simulink library "GTM_aerolib"  (Simulink 7.2)
settings: Solver=ode45  SolverMode=SingleTasking  StartTime=0.0  StopTime=10.0  RelTol=1e-3
undefined symbols (not defined in the file or in its folder): Aero, DamageModels
libraries: simulink_need_slupdate x58, GTM_aerolib x8, simulink x3
(part 3 of 3)

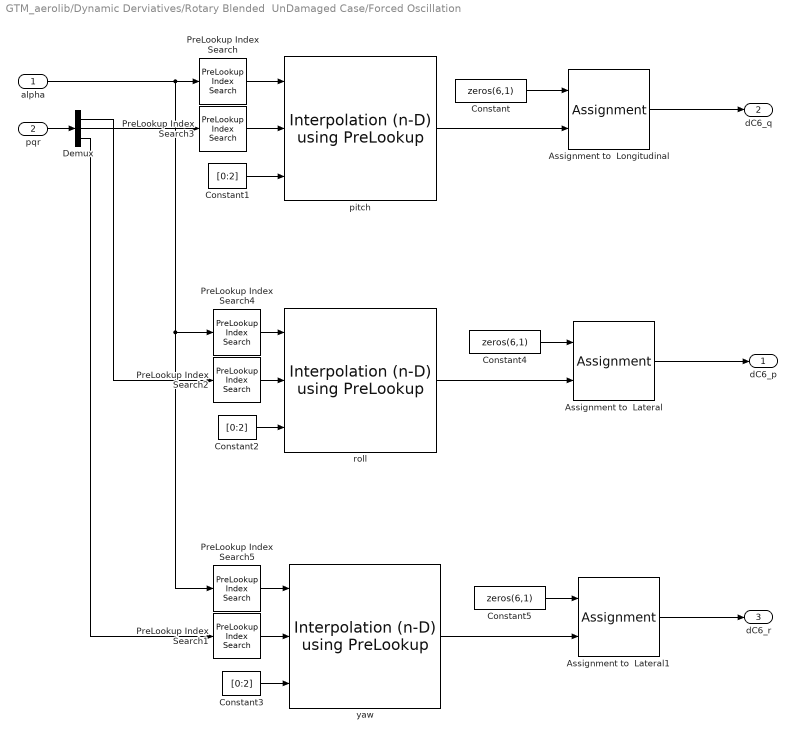
== system GTM_aerolib/Dynamic Derviatives/Rotary Blended  UnDamaged Case/Forced Oscillation ==
  alpha : Inport  OutDataType=sfix(16)  OutScaling=2^0
  pqr : Inport  Port=2  OutDataType=sfix(16)  OutScaling=2^0
  Assignment to  Lateral : Assignment  IndexMode=Zero-based  IndexOptions=Index vector (dialog)  Indices=[1 3 5]  OutputSizes=[1 1]
  Assignment to  Lateral1 : Assignment  IndexMode=Zero-based  IndexOptions=Index vector (dialog)  Indices=[1 3 5]  OutputSizes=[1 1]
  Assignment to  Longitudinal : Assignment  IndexMode=Zero-based  IndexOptions=Index vector (dialog)  Indices=[0 2 4]  OutputSizes=[1 1]
  Constant : Constant  Value=zeros(6,1)  OutDataType=sfix(16)  OutScaling=2^0
  Constant1 : Constant  Value=[0:2]  OutDataTypeMode=uint32  OutDataType=sfix(16)  OutScaling=2^0  OutDataTypeStr=uint32
  Constant2 : Constant  Value=[0:2]  OutDataTypeMode=uint32  OutDataType=sfix(16)  OutScaling=2^0  OutDataTypeStr=uint32
  Constant3 : Constant  Value=[0:2]  OutDataTypeMode=uint32  OutDataType=sfix(16)  OutScaling=2^0  OutDataTypeStr=uint32
  Constant4 : Constant  Value=zeros(6,1)  OutDataType=sfix(16)  OutScaling=2^0
  Constant5 : Constant  Value=zeros(6,1)  OutDataType=sfix(16)  OutScaling=2^0
  Demux : Demux  Outputs=3
  PreLookup Index Search : simulink_need_slupdate/PreLookup Index Search  bpData=Aero.dC3_q.alpha  searchMode=Binary Search  cacheBpFlag=on  outputFlag=off  IndexDataType=uint32  extrapMode=Linear Extrapolation  rangeErrorMode=None
  PreLookup Index Search1 : simulink_need_slupdate/PreLookup Index Search  bpData=Aero.dC3_r.rhat  searchMode=Binary Search  cacheBpFlag=on  outputFlag=off  IndexDataType=uint32  extrapMode=Linear Extrapolation  rangeErrorMode=None
  PreLookup Index Search2 : simulink_need_slupdate/PreLookup Index Search  bpData=Aero.dC3_p.phat  searchMode=Binary Search  cacheBpFlag=on  outputFlag=off  IndexDataType=uint32  extrapMode=Linear Extrapolation  rangeErrorMode=None
  PreLookup Index Search3 : simulink_need_slupdate/PreLookup Index Search  bpData=Aero.dC3_q.qhat  searchMode=Binary Search  cacheBpFlag=on  outputFlag=off  IndexDataType=uint32  extrapMode=Linear Extrapolation  rangeErrorMode=None
  PreLookup Index Search4 : simulink_need_slupdate/PreLookup Index Search  bpData=Aero.dC3_p.alpha  searchMode=Binary Search  cacheBpFlag=on  outputFlag=off  IndexDataType=uint32  extrapMode=Linear Extrapolation  rangeErrorMode=None
  PreLookup Index Search5 : simulink_need_slupdate/PreLookup Index Search  bpData=Aero.dC3_r.alpha  searchMode=Binary Search  cacheBpFlag=on  outputFlag=off  IndexDataType=uint32  extrapMode=Linear Extrapolation  rangeErrorMode=None
  pitch : simulink_need_slupdate/Interpolation (n-D) using PreLookup  numDimsPopupSelect=3  explicitNumDims=2  table=Aero.dC3_q.data  interpMethod=Linear  extrapMethod=Linear  rangeErrorMode=None  NumSelectionDims=1
  roll : simulink_need_slupdate/Interpolation (n-D) using PreLookup  numDimsPopupSelect=3  explicitNumDims=2  table=Aero.dC3_p.data  interpMethod=Linear  extrapMethod=Linear  rangeErrorMode=None  NumSelectionDims=1
  yaw : simulink_need_slupdate/Interpolation (n-D) using PreLookup  numDimsPopupSelect=3  explicitNumDims=2  table=Aero.dC3_r.data  interpMethod=Linear  extrapMethod=Linear  rangeErrorMode=None  NumSelectionDims=1
  dC6_p : Outport  OutDataType=sfix(16)  OutScaling=2^0
  dC6_q : Outport  Port=2  OutDataType=sfix(16)  OutScaling=2^0
  dC6_r : Outport  Port=3  OutDataType=sfix(16)  OutScaling=2^0
  wires:
  PreLookup Index Search5/1 -> yaw/1
  PreLookup Index Search4/1 -> roll/1
  PreLookup Index Search/1 -> pitch/1
  Assignment to  Longitudinal/1 -> dC6_q/1
  Assignment to  Lateral1/1 -> dC6_r/1
  Assignment to  Lateral/1 -> dC6_p/1
  PreLookup Index Search3/1 -> pitch/2
  PreLookup Index Search2/1 -> roll/2
  PreLookup Index Search1/1 -> yaw/2
  yaw/1 -> Assignment to  Lateral1/2
  Constant5/1 -> Assignment to  Lateral1/1
  Constant4/1 -> Assignment to  Lateral/1
  roll/1 -> Assignment to  Lateral/2
  pitch/1 -> Assignment to  Longitudinal/2
  Constant/1 -> Assignment to  Longitudinal/1
  Constant3/1 -> yaw/3
  Constant2/1 -> roll/3
  Demux/3 -> PreLookup Index Search1/1
  Demux/1 -> PreLookup Index Search2/1
  Demux/2 -> PreLookup Index Search3/1
  Constant1/1 -> pitch/3
  pqr/1 -> Demux/1
  alpha/1 -> PreLookup Index Search/1, PreLookup Index Search5/1, PreLookup Index Search4/1

== system GTM_aerolib/Dynamic Derviatives/Rotary Blended  UnDamaged Case/Rotary Balance ==
  alpha : Inport  OutDataType=sfix(16)  OutScaling=2^0
  beta : Inport  Port=2  OutDataType=sfix(16)  OutScaling=2^0
  w : Inport  Port=3  OutDataType=sfix(16)  OutScaling=2^0
  Constant1 : Constant  Value=[0:5]  OutDataTypeMode=uint32  OutDataType=sfix(16)  OutScaling=2^0  OutDataTypeStr=uint32
  PreLookup Index Search : simulink_need_slupdate/PreLookup Index Search  bpData=Aero.dC6_w.alpha  searchMode=Binary Search  cacheBpFlag=on  outputFlag=off  IndexDataType=uint32  extrapMode=Linear Extrapolation  rangeErrorMode=None
  PreLookup Index Search1 : simulink_need_slupdate/PreLookup Index Search  bpData=Aero.dC6_w.beta  searchMode=Binary Search  cacheBpFlag=on  outputFlag=off  IndexDataType=uint32  extrapMode=Linear Extrapolation  rangeErrorMode=None
  PreLookup Index Search2 : simulink_need_slupdate/PreLookup Index Search  bpData=Aero.dC6_w.what  searchMode=Binary Search  cacheBpFlag=on  outputFlag=off  IndexDataType=uint32  extrapMode=Linear Extrapolation  rangeErrorMode=None
  TableLookup : simulink_need_slupdate/Interpolation (n-D) using PreLookup  numDimsPopupSelect=4  explicitNumDims=2  table=Aero.dC6_w.data  interpMethod=Linear  extrapMethod=Linear  rangeErrorMode=None  NumSelectionDims=1
  dC6 : Outport  OutDataType=sfix(16)  OutScaling=2^0
  wires:
  PreLookup Index Search2/1 -> TableLookup/2
  PreLookup Index Search1/1 -> TableLookup/3
  w/1 -> PreLookup Index Search2/1
  Constant1/1 -> TableLookup/4
  TableLookup/1 -> dC6/1
  alpha/1 -> PreLookup Index Search/1
  beta/1 -> PreLookup Index Search1/1
  PreLookup Index Search/1 -> TableLookup/1

== matlab function Control Surfaces/Implement Damage Models/Implement Damage Models ==
  data: SurfVec input double; DamageCase input double; dC6 output double; SurfGain parameter double
function dC6 = fcn(SurfVec,DamageCase,SurfGain)
% This block supports an embeddable subset of the MATLAB language.
% See the help menu for details. 
damagecase = cast(round(DamageCase),'uint32');
Nsurfs=18;
if (damagecase==0),
    dC6=ones(1,Nsurfs)*(reshape(SurfVec,6,Nsurfs)');
else
  gain=squeeze(SurfGain(damagecase,:,:));
  dC6=ones(1,Nsurfs)*( transpose(reshape(SurfVec,6,Nsurfs)).*gain);
end

== matlab function Dynamic Derviatives/Rotary Blended UnDamaged Case/Blending Function ==
  data: alpha input double; omega output double; beta input double; tas input double; pqr input double; pqr_osc output double; B input double; Cbar input double
function[omega,pqr_osc]= hykal(alpha,beta,tas,pqr,B,Cbar)
% Hybrid Kalviste blending method for use in embedded block in Simulink.
%
% Austin Murch
% Austin.M.Murch@nasa.gov

% Dimension vector outputs.
pqr_osc=zeros(3,1);
 

% Constants
dtr=pi/180;
knots2ft=1.689;

% Setup variables
pb=pqr(1);
qb=pqr(2);
rb=pqr(3);

alpha = alpha*dtr;
beta = beta*dtr;
omega = 0;

%----Hybrid Kalviste Method----%
whichcase = 0;

%Test for case 1: p_osc = 0
if cos(alpha)*cos(beta) == 0
elseif pb == 0
else
    omega = pb/(cos(alpha)*cos(beta));
    r_osc = rb - omega*sin(alpha)*cos(beta);
    if abs(r_osc) > abs(rb)
    elseif r_osc*rb < 0
    else
        whichcase = 1;
    end
end

%Test for case 2: r_osc = 0
if sin(alpha)*cos(beta) == 0
elseif rb == 0
else
    omega = rb/(sin(alpha)*cos(beta));
    p_osc = pb - omega*cos(alpha)*cos(beta);
    if abs(p_osc) > abs(pb)
    elseif p_osc*pb < 0
    else
        whichcase = 2;
    end
end

%Test for case 3: Omega = 0
if whichcase == 0
    whichcase = 3;
end

 

switch whichcase
    case 1
        omega = pb/(cos(alpha)*cos(beta));
        pqr_osc(1) = 0;        
        pqr_osc(2) = qb - omega*sin(beta);        
        pqr_osc(3) = rb - omega*sin(alpha)*cos(beta);

    case 2
        omega = rb/(sin(alpha)*cos(beta));
        pqr_osc(1) = pb - omega*cos(alpha)*cos(beta);
        pqr_osc(2) = qb - omega*sin(beta);
        pqr_osc(3) = 0;

    case 3
        pqr_osc(1) = pb;
        pqr_osc(2) = qb;
        pqr_osc(3) = rb;
        omega = 0;
end

%-----------------------------------------------% End Hybrid Kalviste

% Scale values for table lookup
b2vt=B/(2*tas*knots2ft);
c2vt=Cbar/(2*tas*knots2ft);
omega=omega*b2vt;
pqr_osc=pqr_osc.*[b2vt;c2vt;b2vt];
